simulink model "dspintrp"  (Simulink 6.0)
settings: Solver=FixedStepDiscrete  SolverMode=SingleTasking  StartTime=0.0  StopTime=50.0  RelTol=1e-3  AbsTol=1e-6
undefined symbols (not defined in the file or in its folder): intfilt
libraries: dspsigops x1, dspmlti3 x1, dspsrcs4 x1
Description:
  | Interpolation based on multirate filtering.
settings Model: CovMetricSettings=d  Creator=don  LastModifiedBy=sconahan  ExtModeTrigMode=oneshot  ExtModeArmWhenConnect=off
settings DataIOCC: LimitDataPoints=off  SaveOutput=off  SaveTime=off  SignalLoggingName=sigsOut
settings OptimizationCC: BlockReduction=off  BooleanDataType=off  MultiInstanced=off  RollThreshold=2
settings FormatCC: IgnoreBidirectionalLines=off
settings DebuggingCC: SingleTaskRateTransMsg=error  IntegerOverflowMsg=none
settings HardwareCC: TargetUnknown=on
settings CodeAppCC: FileBanners=off  CustomSymbols=off
settings GRTTargetCC: TargetFcnLib=iso_c_tmw.mat  IsERTTarget=off

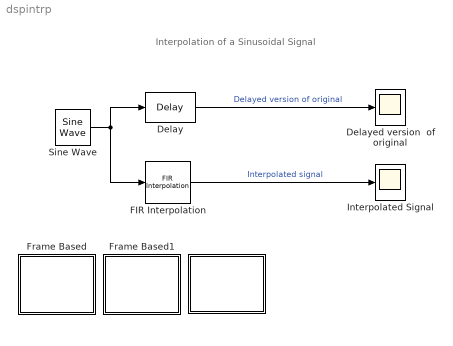
== system dspintrp ==
  note: Interpolation of a Sinusoidal Signal
  " " : Subsystem
      mask Type: Interpolation filter info block
      mask Display: disp('Info')
  Delay : dspsigops/Delay  dly_unit=Samples  delay=9  ic_detail=on  dif_ic_for_ch=off  dif_ic_for_dly=off  ic=0  reset_popup=None
  Delayed version  of original : Scope
      settings: TickLabels=on  YMin=-1.2  YMax=1.2  DataFormat=Array
  FIR Interpolation : dspmlti3/FIR Interpolation  h=intfilt(9, 9, .5)  L=9  framing=Maintain input frame size  outputBufInitCond=0  roundingMode=Floor  overflowMode=off
  Frame Based : Subsystem
      settings: OpenFcn=dspintrpf;
      mask Display: disp('Frame-based\nVersion')
  Frame Based1 : Subsystem
      settings: OpenFcn=dspintrpfp
      mask Display: disp('Fixed-point\nVersion')
  Interpolated Signal : Scope
      settings: TickLabels=on  YMin=-1.2  YMax=1.2  SaveName=ScopeData2  DataFormat=Array
  Sine Wave : dspsrcs4/Sine Wave  Amplitude=1  Frequency=0.2  Phase=0.7  SampleMode=Discrete  OutComplex=Real  CompMethod=Trigonometric fcn  TableSize=Speed  SampleTime=1  SamplesPerFrame=1  dataType=double  wordLen=16  udDataType=sfix(16)  fracBitsMode=Best precision  numFracBits=15  ResetState=Restart at time zero
  wires:
  Sine Wave/1 -> FIR Interpolation/1, Delay/1
  Delay/1 -> Delayed version  of original/1  "Delayed version of original"
  FIR Interpolation/1 -> Interpolated Signal/1  "Interpolated signal"

== system dspintrp/  ==
  note: Interpolation of a Sinusoidal Signal
      |
      | This demo illustrates digital interpolation using an FIR filter.  The DSP Blockset FIR Interpolation
      | block increases the sampling rate of its input signal by a factor of 9.  The interpolated values are
      | calculated by an efficient digital polyphase interpolation filter structure operating at the higher
      | sampling rate.
      |
      | The ideal 9-fold interpolation filter is a lowpass filter, operating at the fast rate 9*fs, with cutoff
      | frequency equal to the low-rate Nyquist frequency fc = fs/2. An FIR approximation to the ideal
      | interpolator is obtained by truncating the ideal impulse response to a finite length, say
      | N = 2*R*L + 1, where R is the upsampling rate (9 in this case) and 2*L is the number of
      | nearest non-zero samples used for interpolation. The 'FIR Interpolation' block uses MATLAB's
      | routine 'intfilt(R,L,ALPHA)' to compute values of the interpolated samples.  Using the
      | polyphase filter implementation, each of the interpolated value , say 'i' (where 0 < i < R-1),
      | is computed by the ith polyphase subfilter, each having length 2*L, acting on L low-rate
      | samples above and L low-rate samples below the desired interpolation time. Using these R
      | subfilters results in a reduced computational cost by a factor of 'R', as compared to using a
      | full, length N interpolation filter.  The original low-rate signal is delayed by 9 samples so as to
      | time-align the original signal and the interpolated one.
      |
      | For more information on the 'FIR interpolation', see S. J. Orfanidis, "Introduction To Signal
      | Processing", Prentice Hall, 1996

== system dspintrp/Frame Based ==

== system dspintrp/Frame Based1 ==
